simulink model "generate_signal"  (R2022b)
settings: Solver=VariableStepAuto  StartTime=0.0  StopTime=2  RelTol=1e-3
undefined symbols (not defined in the file or in its folder): Radix
libraries: commchan3 x2, dspxfrm3 x1, fillib x1
settings Model: NumberOfSteps=100  Creator=Lenovo  LastModifiedBy=Lenovo

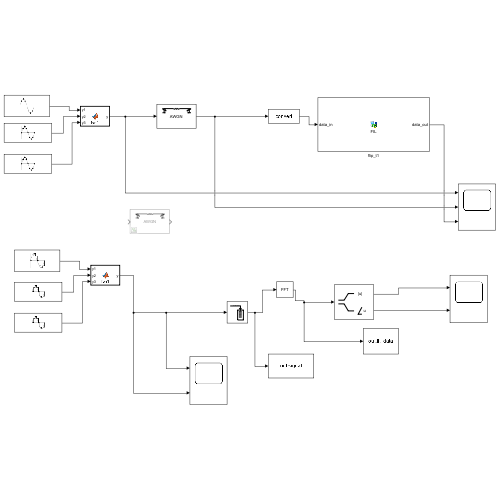
[thumbnail: Simulink's stored preview of the top-level diagram]
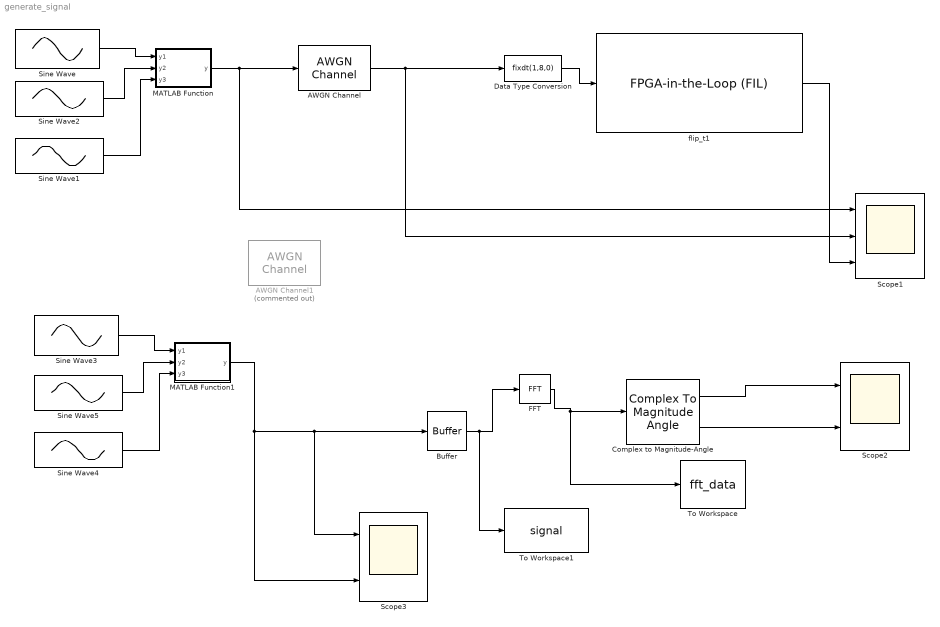
== system generate_signal ==
  AWGN Channel : commchan3/AWGN Channel  InputProcessing=Columns as channels (frame based)  seed=67  noiseMode="Signal to noise ratio  (SNR)"  EbNodB=10  EsNodB=10  SNRdB=-10  bitsPerSym=1  Ps=1  Tsym=1  variance=1
  AWGN Channel1 : commchan3/AWGN Channel  Commented=on  InputProcessing=Columns as channels (frame based)  seed=64  noiseMode="Signal to noise ratio  (SNR)"  EbNodB=10  EsNodB=10  SNRdB=-10  bitsPerSym=1  Ps=1  Tsym=1  variance=1
  Buffer : Buffer  N=1024  OutputFrames=off
  Complex to Magnitude-Angle : ComplexToMagnitudeAngle
  Data Type Conversion : DataTypeConversion  OutMin=[-128]  OutMax=[127]  OutDataTypeStr=fixdt(1,8,0)  RndMeth=Nearest  SaturateOnIntegerOverflow=off
  FFT : dspxfrm3/FFT  FFTImplementation=Radix-2  CompMethod=Table lookup  TableOpt=NEW  TableOptActive=Speed  BitRevOrder=off  Normalize=off  InheritFFTLength=off  FFTLength=1024  WrapInput=off  roundingMode=Nearest  overflowMode=off  firstCoeffDataTypeStr=Inherit: Same word length as input  firstCoeffLastDataTypeStr=Inherit: Same word length as input  outputMin=[]  outputMax=[]
  MATLAB Function : MATLAB Function  TreatAsAtomicUnit=on
  MATLAB Function1 : MATLAB Function  TreatAsAtomicUnit=on
  Scope1 : Scope  NumInputPorts=3
  Scope2 : Scope  NumInputPorts=2
  Scope3 : Scope  NumInputPorts=2
  Sine Wave : Sin  SineType=Sample based  Amplitude=5  Samples=102  SampleTime=1
  Sine Wave1 : Sin  SineType=Sample based  Amplitude=5  Frequency=5  Samples=410  SampleTime=1
  Sine Wave2 : Sin  SineType=Sample based  Amplitude=5  Frequency=5  Samples=205  SampleTime=1
  Sine Wave3 : Sin  Amplitude=100  Frequency=628  Samples=102  SampleTime=0.001
  Sine Wave4 : Sin  Amplitude=100  Frequency=1885  Samples=410  SampleTime=0.001
  Sine Wave5 : Sin  Amplitude=100  Frequency=1257  Samples=205  SampleTime=0.001
  To Workspace : ToWorkspace  VariableName=fft_data  SampleTime=-1
      settings: Save2DSignal=2-D array (concatenate along first dimension)
  To Workspace1 : ToWorkspace  VariableName=signal  SampleTime=-1
      settings: Save2DSignal=2-D array (concatenate along first dimension)
  flip_t1 : fillib/FPGA-in-the-Loop (FIL)  ForceInterfaceUpdate=0.12699
  wires:
  Sine Wave/1 -> MATLAB Function/1(y1)
  Sine Wave2/1 -> MATLAB Function/2(y2)
  MATLAB Function/1(y) -> Scope1/1, AWGN Channel/1
  AWGN Channel/1 -> Scope1/2, Data Type Conversion/1
  Data Type Conversion/1 -> flip_t1/1
  Sine Wave1/1 -> MATLAB Function/3(y3)
  flip_t1/1 -> Scope1/3
  Sine Wave4/1 -> MATLAB Function1/3(y3)
  Sine Wave5/1 -> MATLAB Function1/2(y2)
  Sine Wave3/1 -> MATLAB Function1/1(y1)
  Buffer/1 -> To Workspace1/1, FFT/1
  FFT/1 -> Complex to Magnitude-Angle/1, To Workspace/1
  Complex to Magnitude-Angle/2 -> Scope2/2
  Complex to Magnitude-Angle/1 -> Scope2/1
  MATLAB Function1/1(y) -> Scope3/1, Buffer/1, Scope3/2

== matlab function generate_signal/MATLAB Function ==
  data: y1 input; y output; y2 input; y3 input
function y = fcn1(y1, y2, y3)

y = y1 + y2 + y3;

== matlab function generate_signal/MATLAB Function1 ==
  data: y1 input; y output; y2 input; y3 input
function y = fcn1(y1, y2, y3)

y = y1 + y2 + y3;

y = awgn(y, 10, 'measured');
